simulink subsystem "energy_sizing"  (R2024b)
settings: Solver=VariableStepAuto  StartTime=0.0  StopTime=10.0  RelTol=1e-3
model mask{n_cubes=cubes, vb=v_b, capb=cap}
  mask prompts: n_cubes "Number of cubes to be picked and placed"; vb "Battery voltage (V)"; capb "Cell capacity (Ah)"
settings Model: Creator=Mohammed Hany  LastModifiedBy=Mohammed Hany

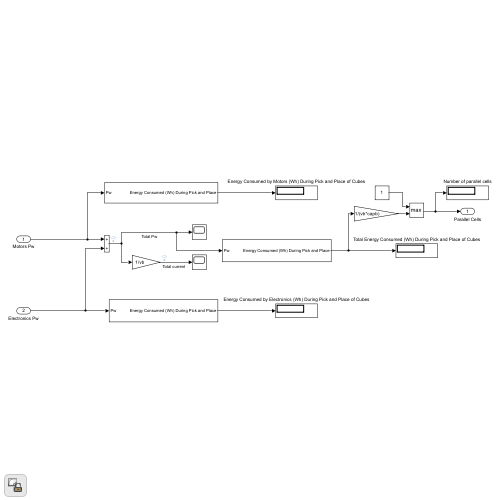
[thumbnail: Simulink's stored preview of the top-level diagram]
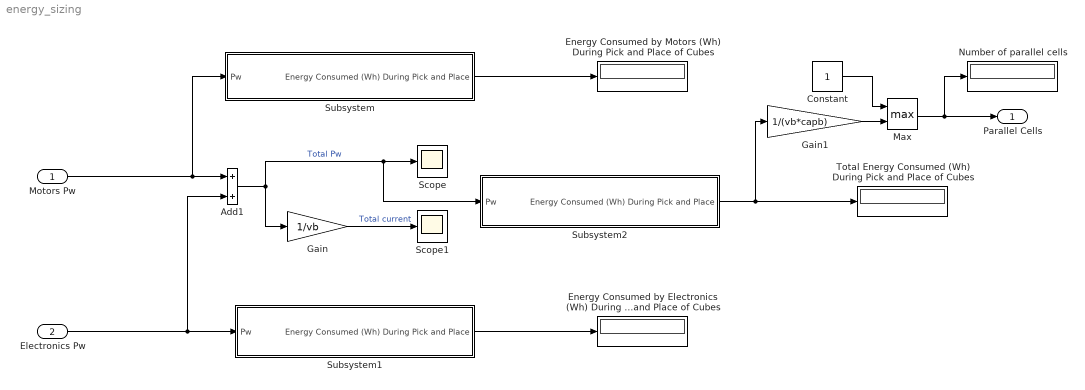
== system energy_sizing ==
  Motors Pw : Inport
  Electronics Pw : Inport  Port=2
  Add1 : Sum
  Constant : Constant
  Energy Consumed by Electronics (Wh) During Pick and Place of Cubes : Display
  Energy Consumed by Motors (Wh) During Pick and Place of Cubes : Display
  Gain : Gain  Gain=1/vb
  Gain1 : Gain  Gain=1/(vb*capb)
  Max : MinMax  Function=max  Inputs=2
  Number of parallel cells : Display
  Scope : Scope
  Scope1 : Scope
  Subsystem : Subsystem  mask{cubes=n_cubes}
      mask prompts: cubes "Number of cubes for pick and place"
  Subsystem1 : Subsystem  mask{cubes=n_cubes}
      mask prompts: cubes "Number of cubes for pick and place"
  Subsystem2 : Subsystem  mask{cubes=n_cubes}
      mask prompts: cubes "Number of cubes for pick and place"
  Total Energy Consumed (Wh) During Pick and Place of Cubes : Display
  Parallel Cells : Outport
  wires:
  Gain/1 -> Scope1/1  "Total current"
  Motors Pw/1 -> Add1/1, Subsystem/1(Pw)
  Electronics Pw/1 -> Subsystem1/1(Pw), Add1/2
  Subsystem/1(Energy Consumed (Wh) During Pick and Place) -> Energy Consumed by Motors (Wh) During Pick and Place of Cubes/1
  Add1/1 -> Scope/1, Subsystem2/1(Pw), Gain/1  "Total Pw"
  Subsystem1/1(Energy Consumed (Wh) During Pick and Place) -> Energy Consumed by Electronics (Wh) During Pick and Place of Cubes/1
  Subsystem2/1(Energy Consumed (Wh) During Pick and Place) -> Total Energy Consumed (Wh) During Pick and Place of Cubes/1, Gain1/1
  Gain1/1 -> Max/2
  Constant/1 -> Max/1
  Max/1 -> Parallel Cells/1, Number of parallel cells/1

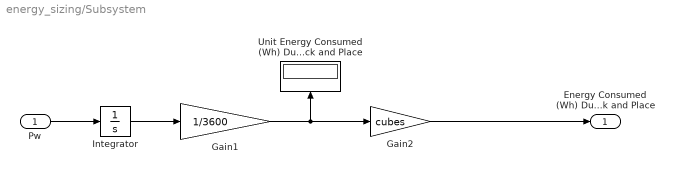
== system energy_sizing/Subsystem ==
  Pw : Inport
  Gain1 : Gain  Gain=1/3600
  Gain2 : Gain  Gain=cubes
  Integrator : Integrator
  Unit Energy Consumed (Wh) During Pick and Place : Display
  Energy Consumed (Wh) During Pick and Place : Outport
  wires:
  Pw/1 -> Integrator/1
  Gain2/1 -> Energy Consumed (Wh) During Pick and Place/1
  Gain1/1 -> Unit Energy Consumed (Wh) During Pick and Place/1, Gain2/1
  Integrator/1 -> Gain1/1

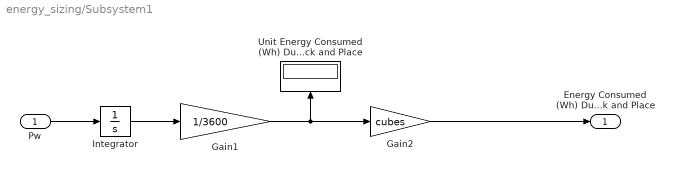
== system energy_sizing/Subsystem1 ==
  Pw : Inport
  Gain1 : Gain  Gain=1/3600
  Gain2 : Gain  Gain=cubes
  Integrator : Integrator
  Unit Energy Consumed (Wh) During Pick and Place : Display
  Energy Consumed (Wh) During Pick and Place : Outport
  wires:
  Pw/1 -> Integrator/1
  Gain2/1 -> Energy Consumed (Wh) During Pick and Place/1
  Gain1/1 -> Unit Energy Consumed (Wh) During Pick and Place/1, Gain2/1
  Integrator/1 -> Gain1/1

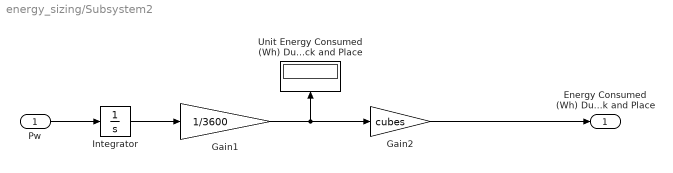
== system energy_sizing/Subsystem2 ==
  Pw : Inport
  Gain1 : Gain  Gain=1/3600
  Gain2 : Gain  Gain=cubes
  Integrator : Integrator
  Unit Energy Consumed (Wh) During Pick and Place : Display
  Energy Consumed (Wh) During Pick and Place : Outport
  wires:
  Pw/1 -> Integrator/1
  Gain2/1 -> Energy Consumed (Wh) During Pick and Place/1
  Gain1/1 -> Unit Energy Consumed (Wh) During Pick and Place/1, Gain2/1
  Integrator/1 -> Gain1/1
